simulink model "Modelo_Red_Mitigación_final"  (R2019b)
settings: Solver=VariableStepAuto  StartTime=0.0  StopTime=2.5  RelTol=1e-3
InitFcn:
  | Ts=20e-6;
undefined symbols (not defined in the file): D1, Delta, Ion, Lithium
libraries: powerlib x371, powerlib_meascontrol x286, simulink x50, simulink_extras x20, electricdrivelib x16
(part 7 of 11)

== system Modelo_Red_Mitigación_final/Modelo bateria pasiva/Subsystem3/Subsystem2 ==
  AC_CONTROL ALGORITHM : Subsystem
  Battery : electricdrivelib/Extra Sources/Battery  Commented=on  BatType=Lithium-Ion  ShowTempParam=off  ThermalPreset=no  ShowAgeParam=off  NomV=2000  NomQ=2  SOC=100  Batt_Tr=2  PresetModel=on  MaxQ=2  MinV=1500  FullV=2327.9743  Dis_rate=0.86957  R=10  Normal_OP=1.8087  expZone="[2160.7717     0.09826087]"  current=[0.2 0.4 1]  Units=Time  Tci=20  NomT=20  T2=-30  MaxQ2=4.8  FullV2=7.1  Normal_OP2=5.655  expZone2="[6.58           1]"  Rca=0.6  ti=2000  Dp=0  Neq0=0  Tsim=1e6  Ta1=25  Qeol=5.4*0.9  Reol=0.013333*1.2  Char_age=[2000, 3000]  Dis_age=[2000, 3000]  N1=1500  N2=10500  N3=1000  N4=1400  Ta2=45  N5=950
      settings: SourceProductName=Simscape Electrical
  Battery1 : electricdrivelib/Extra Sources/Battery  BatType=Lithium-Ion  ShowTempParam=off  ThermalPreset=no  ShowAgeParam=off  NomV=1800  NomQ=200  SOC=100  Batt_Tr=20  PresetModel=off  MaxQ=1  MinV=1500  FullV=2000  Dis_rate=5  R=0.1  Normal_OP=1  expZone="[1960.7717       0.9826087]"  current=[6.5 13 200]  Units=Time  Tci=20  NomT=20  T2=25  MaxQ2=200  FullV2=2000  Normal_OP2=1500  expZone2="[2160.7717       9.826087]"  Rca=0.6411  ti=4880  Dp=0  Neq0=0  Tsim=1e6  Ta1=25  Qeol=5.4*0.9  Reol=0.013333*1.2  Char_age=[2.3478, 3]  Dis_age=[2.3478, 10]  N1=1500  N2=10500  N3=1000  N4=1400  Ta2=45  N5=950
      settings: SourceProductName=Simscape Electrical
  Bus Selector : BusSelector  OutputSignals=SOC (%),Current (A),Voltage (V)
  Control1 : Subsystem
  "Control1 " : Subsystem  Commented=on
  Control2 : Subsystem  Commented=on
  Current Measurement1 : powerlib/Measurements/Current Measurement  PhasorSimulation=off  OutputType=Complex  PSBequivalent=0
      settings: SourceProductName=Simscape Electrical
  Current Measurement3 : powerlib/Measurements/Current Measurement  PhasorSimulation=off  OutputType=Complex  PSBequivalent=0
      settings: SourceProductName=Simscape Electrical
  Currents : Scope  NumInputPorts=2
  First-Order Filter3 : powerlib_meascontrol/Filters/First-Order Filter  FilterType=Lowpass  Tc=10e-3  Ts=0  Initialize=on  Vac_Init=[0, 0, 60]  Vdc_Init=0  PlotResponse=off  FreqRange="[0,  200,  1]"
      settings: SourceProductName=Simscape Electrical
  First-Order Filter4 : powerlib_meascontrol/Filters/First-Order Filter  FilterType=Lowpass  Tc=10e-3  Ts=0  Initialize=on  Vac_Init=[0, 0, 60]  Vdc_Init=0  PlotResponse=off  FreqRange="[0,  200,  1]"
      settings: SourceProductName=Simscape Electrical
  Half-Bridge Converter : powerlib/Power Electronics/Half-Bridge Converter  Commented=on  ModelType=Switching devices  Ron=1e-3  Rs=1e6  Cs=inf  Vforward=[0,0]  Ron_Diode=1e-3  Rs_Diode=1e6  Cs_Diode=inf  Vf_Diode=1e-3  Rs_CurrentSource=inf
      settings: SourceProductName=Simscape Electrical  SourceProductBaseCode=PS
  P SC in 1 : Scope
  "Power (3ph, Instantaneous)2" : powerlib_meascontrol/Measurements/Power (3ph, Instantaneous)
      settings: SourceProductName=Simscape Electrical
  Q Sc in 1 : Scope
  Series RLC Branch1 : powerlib/Elements/Series RLC Branch  LConnTagsString=__new0  RConnTagsString=__new0  BranchType=R  Resistance=0.1  Inductance=1e-3  SetiL0=off  InitialCurrent=0  Capacitance=220e-6  Setx0=off  InitialVoltage=0  Measurements=None
      settings: SourceProductName=Simscape Electrical
  Series RLC Branch2 : powerlib/Elements/Series RLC Branch  LConnTagsString=__new0  RConnTagsString=__new0  BranchType=C  Resistance=10e6  Inductance=1e-3  SetiL0=off  InitialCurrent=0  Capacitance=220e-6  Setx0=off  InitialVoltage=0  Measurements=None
      settings: SourceProductName=Simscape Electrical
  Series RLC Branch3 : powerlib/Elements/Series RLC Branch  LConnTagsString=__new0  RConnTagsString=__new0  BranchType=R  Resistance=0.5  Inductance=1e-3  SetiL0=off  InitialCurrent=0  Capacitance=220e-6  Setx0=off  InitialVoltage=0  Measurements=None
      settings: SourceProductName=Simscape Electrical
  Three-Phase V-I Measurement1 : powerlib/Measurements/Three-Phase V-I Measurement  VoltageMeasurement=phase-to-phase  SetLabelV=on  LabelV=Vabc_SC2  Vpu=off  VpuLL=off  CurrentMeasurement=yes  SetLabelI=on  LabelI=Iabc_SC2  Ipu=off  Pbase=100e6  Vbase=500e3  OutputType=Complex  PhasorSimulation=off  PSBequivalent=0
      settings: SourceProductName=Simscape Electrical
  To Workspace : ToWorkspace  VariableName=datosbatpasiva  SaveFormat=Timeseries  SampleTime=1E-5
  Two-Level Converter1 : powerlib/Power Electronics/Two-Level Converter  ModelType=Average model (Uref-controlled)  Ron=1e-3  Rs=1e6  Cs=inf  Vforward=[0,0]  Ron_Diode=1e-3  Rs_Diode=1e6  Cs_Diode=inf  Vf_Diode=1e-3  Rs_CurrentSource=inf
      settings: SourceProductName=Simscape Electrical  SourceProductBaseCode=PS
  V DC : Scope  NumInputPorts=2
  Variables SC1 : Scope  NumInputPorts=3
  VinvSC : Scope  NumInputPorts=2
  Voltage Measurement : powerlib/Measurements/Voltage Measurement  PhasorSimulation=off  OutputType=Complex  PSBequivalent=0
      settings: SourceProductName=Simscape Electrical
  A : PMIOPort  Side=Left
  B : PMIOPort  Port=2  Side=Left
  C : PMIOPort  Port=3  Side=Left
  tag scope: Iload=global, Vdc=global
  wires:
  [Iobat] -> Currents/2
  [Ibat] -> Currents/1  "Ibatout"
  Voltage Measurement/1 -> [Vdc]
  Current Measurement1/1 -> [Iload]
  Current Measurement3/1 -> [Iobat]
  [IoutConv] -> V DC/2
  [Vdc] -> V DC/1
  [Uref] -> Two-Level Converter1/1
  [Vabc_SC2] -> VinvSC/1
  "Power (3ph, Instantaneous)2"/1 -> First-Order Filter3/1
  First-Order Filter4/1 -> Q Sc in 1/1
  [Vabc_SC2] -> "Power (3ph, Instantaneous)2"/1
  First-Order Filter3/1 -> P SC in 1/1
  [Iabc_SC2] -> "Power (3ph, Instantaneous)2"/2
  "Power (3ph, Instantaneous)2"/2 -> First-Order Filter4/1
  Battery1/1 -> Bus Selector/1, To Workspace/1
  Bus Selector/1 -> Variables SC1/1  "<SOC (%)>"
  Bus Selector/3 -> Variables SC1/3  "<Voltage (V)>"
  Bus Selector/2 -> Variables SC1/2  "<Current (A)>"
  connections:
  Voltage Measurement/LConn1 -- Current Measurement3/RConn1 -- Series RLC Branch2/LConn1 -- Current Measurement1/LConn1
  Current Measurement1/RConn1 -- Two-Level Converter1/RConn1
  A/RConn1 -- Three-Phase V-I Measurement1/LConn1
  C/RConn1 -- Three-Phase V-I Measurement1/LConn3
  B/RConn1 -- Three-Phase V-I Measurement1/LConn2
  Three-Phase V-I Measurement1/RConn1 -- Two-Level Converter1/LConn1
  Three-Phase V-I Measurement1/RConn2 -- Two-Level Converter1/LConn2
  Three-Phase V-I Measurement1/RConn3 -- Two-Level Converter1/LConn3
  Voltage Measurement/LConn2 -- Battery1/LConn2 -- Series RLC Branch3/RConn1 -- Two-Level Converter1/RConn2 -- Series RLC Branch2/RConn1
  Series RLC Branch1/LConn1 -- Current Measurement3/LConn1
  Series RLC Branch1/RConn1 -- Battery1/LConn1 -- Series RLC Branch3/LConn1

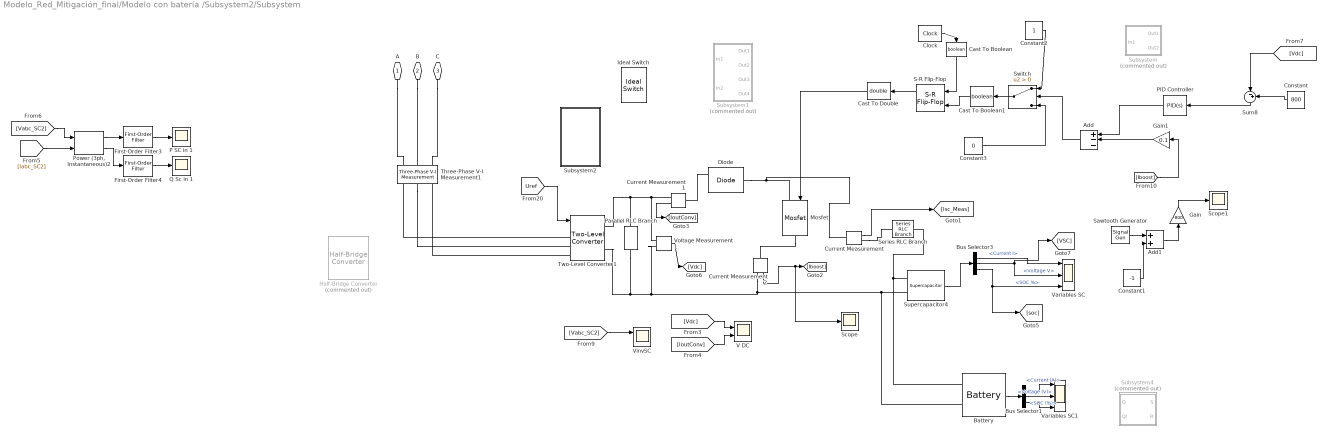
== system Modelo_Red_Mitigación_final/Modelo con batería /Subsystem2/Subsystem ==
  Add : Sum  Inputs=+--
  Add1 : Sum
  Battery : electricdrivelib/Extra Sources/Battery  BatType=Lithium-Ion  ShowTempParam=off  ThermalPreset=no  ShowAgeParam=off  NomV=500  NomQ=500  SOC=100  Batt_Tr=30  PresetModel=on  MaxQ=500  MinV=375  FullV=581.9936  Dis_rate=217.3913  R=0.01  Normal_OP=452.1739  expZone="[540.1929      24.56522]"  current=[6.5 13 32.5]  Units=Time  Tci=20  NomT=20  T2=-30  MaxQ2=4.8  FullV2=7.1  Normal_OP2=5.655  expZone2="[6.58           1]"  Rca=0.6  ti=2000  Dp=0  Neq0=0  Tsim=1e6  Ta1=25  Qeol=5.4*0.9  Reol=0.013333*1.2  Char_age=[2.3478, 3]  Dis_age=[2.3478, 10]  N1=1500  N2=10500  N3=1000  N4=1400  Ta2=45  N5=950
      settings: SourceProductName=Simscape Electrical
  Bus Selector1 : BusSelector  OutputSignals=Current (A),Voltage (V),SOC (%)
  Bus Selector3 : BusSelector  OutputSignals=Current I,Voltage V,SOC %
  Cast To Boolean : DataTypeConversion  OutDataTypeStr=boolean
  Cast To Boolean1 : DataTypeConversion  OutDataTypeStr=boolean
  Cast To Double : DataTypeConversion  OutDataTypeStr=double
  Clock : simulink_extras/Flip Flops/Clock  period=1/10e3
  Constant : Constant  Value=800
  Constant1 : Constant  Value=-1
  Constant2 : Constant
  Constant3 : Constant  Value=0
  Current Measurement : powerlib/Measurements/Current Measurement  PhasorSimulation=off  OutputType=Complex  PSBequivalent=0
      settings: SourceProductName=Simscape Electrical
  Current Measurement1 : powerlib/Measurements/Current Measurement  PhasorSimulation=off  OutputType=Complex  PSBequivalent=0
      settings: SourceProductName=Simscape Electrical
  Current Measurement2 : powerlib/Measurements/Current Measurement  PhasorSimulation=off  OutputType=Complex  PSBequivalent=0
      settings: SourceProductName=Simscape Electrical
  Diode : powerlib/Power Electronics/Diode  Ron=0.001  Lon=0  Vf=0.8  IC=0  UseSnubber=0  Rs=500  Cs=250e-9  Measurements=on
      settings: SourceProductName=Simscape Electrical
  First-Order Filter3 : powerlib_meascontrol/Filters/First-Order Filter  FilterType=Lowpass  Tc=10e-3  Ts=0  Initialize=on  Vac_Init=[0, 0, 60]  Vdc_Init=0  PlotResponse=off  FreqRange="[0,  200,  1]"
      settings: SourceProductName=Simscape Electrical
  First-Order Filter4 : powerlib_meascontrol/Filters/First-Order Filter  FilterType=Lowpass  Tc=10e-3  Ts=0  Initialize=on  Vac_Init=[0, 0, 60]  Vdc_Init=0  PlotResponse=off  FreqRange="[0,  200,  1]"
      settings: SourceProductName=Simscape Electrical
  Gain : Gain  Gain=-800
  Gain1 : Gain  Gain=0.1
  Half-Bridge Converter : powerlib/Power Electronics/Half-Bridge Converter  Commented=on  ModelType=Switching devices  Ron=1e-3  Rs=1e6  Cs=inf  Vforward=[0,0]  Ron_Diode=1e-3  Rs_Diode=1e6  Cs_Diode=inf  Vf_Diode=1e-3  Rs_CurrentSource=inf
      settings: SourceProductName=Simscape Electrical  SourceProductBaseCode=PS
  Ideal Switch : powerlib/Power Electronics/Ideal Switch  Ron=1e-3  Lon=0  IC=1  Rs=1e5  Cs=inf  Measurements=on
      settings: SourceProductName=Simscape Electrical
  Mosfet : powerlib/Power Electronics/Mosfet  Ron=0.1  Lon=0  Rd=0.01  Vfd=0  IC=0  Rs=1e5  Cs=inf  Measurements=off
      settings: SourceProductName=Simscape Electrical
  P SC in 1 : Scope
  PID Controller : simulink/Continuous/PID Controller  Controller=PID  Form=Parallel  TimeDomain=Continuous-time  SampleTime=-1  IntegratorMethod=Forward Euler  FilterMethod=Forward Euler  ControllerParametersSource=internal  P=40  I=10  D=0  UseFilter=on  N=100  TunerSelectOption=Transfer Function Based (PID Tuner App)  InitialConditionSource=internal  InitialConditionForIntegrator=0  InitialConditionForFilter=0  DifferentiatorICPrevScaledInput=0  ExternalReset=none  TrackingMode=off  Kt=1  LimitOutput=off  UpperSaturationLimit=inf  LowerSaturationLimit=-inf  LinearizeAsGain=on  AntiWindupMode=none  Kb=1  POutMin=[]  POutMax=[]  IOutMin=[]  IOutMax=[]  DOutMin=[]  DOutMax=[]  NOutMin=[]  NOutMax=[]  SumOutMin=[]  SumOutMax=[]  SaturationOutMin=[]  SaturationOutMax=[]  PParamMin=[]  PParamMax=[]  IParamMin=[]  IParamMax=[]  DParamMin=[]  DParamMax=[]  NParamMin=[]  NParamMax=[]  KbParamMin=[]  KbParamMax=[]  KtParamMin=[]  KtParamMax=[]  KbOutMin=[]  KbOutMax=[]  KtOutMin=[]  KtOutMax=[]  IntegratorOutMin=[]  IntegratorOutMax=[]  FilterOutMin=[]  FilterOutMax=[]  SumI1OutMin=[]  SumI1OutMax=[]  SumI2OutMin=[]  SumI2OutMax=[]  SumI3OutMin=[]  SumI3OutMax=[]  SumI4OutMin=[]  SumI4OutMax=[]  SumDOutMin=[]  SumDOutMax=[]  DifferentiatorOutMin=[]  DifferentiatorOutMax=[]  FilterDiffOutCoefMin=[]  FilterDiffOutCoefMax=[]  ReciprocalOutMin=[]  ReciprocalOutMax=[]  SumDenOutMin=[]  SumDenOutMax=[]  SumNumOutMin=[]  SumNumOutMax=[]  DivideOutMin=[]  DivideOutMax=[]  IntegratorContinuousStateAttributes=''  IntegratorStateMustResolveToSignalObject=off  IntegratorRTWStateStorageClass=Auto  FilterContinuousStateAttributes=''  FilterStateMustResolveToSignalObject=off  FilterRTWStateStorageClass=Auto  ParallelPVariant=InternalParameters  IdealPVariant=Disabled  IVariant=InternalParameters  DVariant=InternalParameters  IntegratorVariant=Continuous  SatVariant=Disabled  AWVariant=Passthrough  PCopyVariant=Disabled  TRVariant=Disabled  FdbkBlocksVariant=Forward  IdealPFdbkVariant=Disabled  SatFdbkVariant=Disabled  DerivativeFilterVariant=ContFilter  NVariant=InternalParameters  NCopyVariant=Disabled  FilterICVariant=InternalICsFilter  IntegratorICVariant=InternalICs  ExternalResetVariant=Disabled  TRSumVariant=Passthrough  SumFdbkVariant=Disabled  SumVariant=Sum_PID
  Parallel RLC Branch : powerlib/Elements/Parallel RLC Branch  LConnTagsString=a  RConnTagsString=__new0  BranchType=C  Resistance=0.01  Inductance=1e-3  SetiL0=off  InitialCurrent=0  Capacitance=6600e-6  Setx0=off  InitialVoltage=800  Measurements=None
      settings: SourceProductName=Simscape Electrical
  "Power (3ph, Instantaneous)2" : powerlib_meascontrol/Measurements/Power (3ph, Instantaneous)
      settings: SourceProductName=Simscape Electrical
  Q Sc in 1 : Scope
  S-R Flip-Flop : simulink_extras/Flip Flops/S-R Flip-Flop  initial_condition=1
  Sawtooth Generator : SignalGenerator  WaveForm=sawtooth  Frequency=10e3
  Scope : Scope
  Scope1 : Scope
  Series RLC Branch : powerlib/Elements/Series RLC Branch  LConnTagsString=__new0  RConnTagsString=__new0  BranchType=L  Resistance=65e-3  Inductance=1e-3  SetiL0=off  InitialCurrent=0  Capacitance=1e-6  Setx0=off  InitialVoltage=0  Measurements=None
      settings: SourceProductName=Simscape Electrical
  Subsystem : Subsystem  Commented=on
  Subsystem1 : Subsystem  Commented=on
  Subsystem2 : Subsystem
  Subsystem4 : Subsystem  Commented=on
  Sum8 : Sum  Inputs=|-+
  Supercapacitor4 : electricdrivelib/Extra Sources/Supercapacitor  C=18  Rdc=7e-3  Voltage=500  Ns=1  Np=1  Vinit=500  Temp=25  PresetModel=on  EstParam=off  Nc=1  r=1e-9  epsilon=6.0208e-10  Ich=10  Vstern="[0.161  2.7  7.8]"  Self_dis=off  Ioc=10  Vself="[48  47.8  47.06  44.65]"  demandeplot=off  I="[10  20 100  500]"  Units=sec  Vmax=0  If=0  deltaV=0  alpha=0  sec=0
      settings: SourceProductName=Simscape Electrical  SourceProductBaseCode=PS
  Switch : Switch  Criteria=u2 > Threshold
  Three-Phase V-I Measurement1 : powerlib/Measurements/Three-Phase V-I Measurement  VoltageMeasurement=phase-to-phase  SetLabelV=on  LabelV=Vabc_SC2  Vpu=off  VpuLL=off  CurrentMeasurement=yes  SetLabelI=on  LabelI=Iabc_SC2  Ipu=off  Pbase=100e6  Vbase=500e3  OutputType=Complex  PhasorSimulation=off  PSBequivalent=0
      settings: SourceProductName=Simscape Electrical
  Two-Level Converter1 : powerlib/Power Electronics/Two-Level Converter  ModelType=Average model (Uref-controlled)  Ron=1e-3  Rs=1e6  Cs=inf  Vforward=[0,0]  Ron_Diode=1e-3  Rs_Diode=1e6  Cs_Diode=inf  Vf_Diode=1e-3  Rs_CurrentSource=inf
      settings: SourceProductName=Simscape Electrical  SourceProductBaseCode=PS
  V DC : Scope  NumInputPorts=2
  Variables SC : Scope  NumInputPorts=3
  Variables SC1 : Scope  NumInputPorts=3
  VinvSC : Scope  NumInputPorts=2
  Voltage Measurement1 : powerlib/Measurements/Voltage Measurement  PhasorSimulation=off  OutputType=Complex  PSBequivalent=0
      settings: SourceProductName=Simscape Electrical
  A : PMIOPort  Side=Left
  B : PMIOPort  Port=2  Side=Left
  C : PMIOPort  Port=3  Side=Left
  wires:
  Current Measurement/1 -> [Isc_Meas]
  Bus Selector3/2 -> Variables SC/2, [VSC]  "<Voltage V>"
  Bus Selector3/3 -> [soc], Variables SC/3  "<SOC %>"
  Bus Selector3/1 -> Variables SC/1  "<Current I>"
  "Power (3ph, Instantaneous)2"/2 -> First-Order Filter4/1
  [Iabc_SC2] -> "Power (3ph, Instantaneous)2"/2
  First-Order Filter3/1 -> P SC in 1/1
  [Vabc_SC2] -> "Power (3ph, Instantaneous)2"/1
  First-Order Filter4/1 -> Q Sc in 1/1
  "Power (3ph, Instantaneous)2"/1 -> First-Order Filter3/1
  [Vabc_SC2] -> VinvSC/1
  Voltage Measurement1/1 -> [Vdc]
  [Uref] -> Two-Level Converter1/1
  Current Measurement1/1 -> [IoutConv]
  [Vdc] -> V DC/1
  [IoutConv] -> V DC/2
  Supercapacitor4/1 -> Bus Selector3/1
  Current Measurement2/1 -> Scope/1, [Iboost]
  [Iboost] -> Gain1/1
  Constant/1 -> Sum8/2
  [Vdc] -> Sum8/1
  Cast To Boolean1/1 -> S-R Flip-Flop/2
  Cast To Double/1 -> Mosfet/1
  Clock/1 -> Cast To Boolean/1
  Add/1 -> Switch/2
  Cast To Boolean/1 -> S-R Flip-Flop/1
  S-R Flip-Flop/1 -> Cast To Double/1
  Constant3/1 -> Switch/3
  Switch/1 -> Cast To Boolean1/1
  Constant2/1 -> Switch/1
  Sum8/1 -> PID Controller/1
  Bus Selector1/2 -> Variables SC1/2  "<Voltage (V)>"
  Battery/1 -> Bus Selector1/1
  Bus Selector1/3 -> Variables SC1/3  "<SOC (%)>"
  Bus Selector1/1 -> Variables SC1/1  "<Current (A)>"
  Gain1/1 -> Add/2
  PID Controller/1 -> Add/1
  Sawtooth Generator/1 -> Add1/1
  Add1/1 -> Gain/1
  Constant1/1 -> Add1/2
  Gain/1 -> Scope1/1
  connections:
  Current Measurement/RConn1 -- Series RLC Branch/LConn1
  Voltage Measurement1/LConn2 -- Battery/LConn2 -- Supercapacitor4/LConn2 -- Current Measurement2/RConn1 -- Two-Level Converter1/RConn2 -- Parallel RLC Branch/RConn1
  B/RConn1 -- Three-Phase V-I Measurement1/LConn2
  C/RConn1 -- Three-Phase V-I Measurement1/LConn3
  A/RConn1 -- Three-Phase V-I Measurement1/LConn1
  Parallel RLC Branch/LConn1 -- Two-Level Converter1/RConn1 -- Current Measurement1/RConn1 -- Voltage Measurement1/LConn1
  Diode/LConn1 -- Mosfet/LConn1 -- Current Measurement/LConn1
  Two-Level Converter1/LConn1 -- Three-Phase V-I Measurement1/RConn1
  Three-Phase V-I Measurement1/RConn2 -- Two-Level Converter1/LConn2
  Two-Level Converter1/LConn3 -- Three-Phase V-I Measurement1/RConn3
  Mosfet/RConn1 -- Current Measurement2/LConn1
  Diode/RConn1 -- Current Measurement1/LConn1
  Supercapacitor4/LConn1 -- Battery/LConn1 -- Series RLC Branch/RConn1

== system Modelo_Red_Mitigación_final/Modelo con batería /Subsystem3/Subsystem2 ==
  AC_CONTROL ALGORITHM : Subsystem
  Battery : electricdrivelib/Extra Sources/Battery  BatType=Lithium-Ion  ShowTempParam=off  ThermalPreset=no  ShowAgeParam=off  NomV=1000  NomQ=10  SOC=80  Batt_Tr=2  PresetModel=on  MaxQ=10  MinV=750  FullV=1163.9871  Dis_rate=4.3478  R=1  Normal_OP=9.0435  expZone="[1080.3859     0.49130435]"  current=[0.2 0.4 1]  Units=Time  Tci=20  NomT=20  T2=-30  MaxQ2=4.8  FullV2=7.1  Normal_OP2=5.655  expZone2="[6.58           1]"  Rca=0.6  ti=2000  Dp=0  Neq0=0  Tsim=1e6  Ta1=25  Qeol=5.4*0.9  Reol=0.013333*1.2  Char_age=[2000, 3000]  Dis_age=[2000, 3000]  N1=1500  N2=10500  N3=1000  N4=1400  Ta2=45  N5=950
      settings: SourceProductName=Simscape Electrical
  Bus Selector1 : BusSelector  OutputSignals=Current (A),Voltage (V),SOC (%)
  Control1 : Subsystem
  "Control1 " : Subsystem  Commented=on
  Control2 : Subsystem  Commented=on
  Current Measurement1 : powerlib/Measurements/Current Measurement  PhasorSimulation=off  OutputType=Complex  PSBequivalent=0
      settings: SourceProductName=Simscape Electrical
  Current Measurement2 : powerlib/Measurements/Current Measurement  PhasorSimulation=off  OutputType=Complex  PSBequivalent=0
      settings: SourceProductName=Simscape Electrical
  Current Measurement3 : powerlib/Measurements/Current Measurement  PhasorSimulation=off  OutputType=Complex  PSBequivalent=0
      settings: SourceProductName=Simscape Electrical
  Currents : Scope  NumInputPorts=2
  First-Order Filter3 : powerlib_meascontrol/Filters/First-Order Filter  FilterType=Lowpass  Tc=10e-3  Ts=0  Initialize=on  Vac_Init=[0, 0, 60]  Vdc_Init=0  PlotResponse=off  FreqRange="[0,  200,  1]"
      settings: SourceProductName=Simscape Electrical
  First-Order Filter4 : powerlib_meascontrol/Filters/First-Order Filter  FilterType=Lowpass  Tc=10e-3  Ts=0  Initialize=on  Vac_Init=[0, 0, 60]  Vdc_Init=0  PlotResponse=off  FreqRange="[0,  200,  1]"
      settings: SourceProductName=Simscape Electrical
  Ground : powerlib/Elements/Ground  LConnTagsString=a
      settings: SourceProductName=Simscape Electrical
  Half-Bridge Converter : powerlib/Power Electronics/Half-Bridge Converter  Commented=on  ModelType=Switching devices  Ron=1e-3  Rs=1e6  Cs=inf  Vforward=[0,0]  Ron_Diode=1e-3  Rs_Diode=1e6  Cs_Diode=inf  Vf_Diode=1e-3  Rs_CurrentSource=inf
      settings: SourceProductName=Simscape Electrical  SourceProductBaseCode=PS
  Half-Bridge Converter2 : powerlib/Power Electronics/Half-Bridge Converter  ModelType=Switching devices  Ron=1e-3  Rs=1e6  Cs=inf  Vforward=[0,0]  Ron_Diode=1e-3  Rs_Diode=1e6  Cs_Diode=inf  Vf_Diode=1e-3  Rs_CurrentSource=inf
      settings: SourceProductName=Simscape Electrical  SourceProductBaseCode=PS
  P SC in 1 : Scope
  Parallel RLC Branch : powerlib/Elements/Parallel RLC Branch  LConnTagsString=a  RConnTagsString=__new0  BranchType=C  Resistance=0.01  Inductance=1e-3  SetiL0=off  InitialCurrent=0  Capacitance=220e-6  Setx0=on  InitialVoltage=1500  Measurements=None
      settings: SourceProductName=Simscape Electrical
  "Power (3ph, Instantaneous)2" : powerlib_meascontrol/Measurements/Power (3ph, Instantaneous)
      settings: SourceProductName=Simscape Electrical
  Q Sc in 1 : Scope
  Series RLC Branch1 : powerlib/Elements/Series RLC Branch  LConnTagsString=__new0  RConnTagsString=__new0  BranchType=L  Resistance=65e-3  Inductance=1.67e-3  SetiL0=off  InitialCurrent=0  Capacitance=1e-6  Setx0=off  InitialVoltage=0  Measurements=None
      settings: SourceProductName=Simscape Electrical
  Three-Phase V-I Measurement1 : powerlib/Measurements/Three-Phase V-I Measurement  VoltageMeasurement=phase-to-phase  SetLabelV=on  LabelV=Vabc_SC2  Vpu=off  VpuLL=off  CurrentMeasurement=yes  SetLabelI=on  LabelI=Iabc_SC2  Ipu=off  Pbase=100e6  Vbase=500e3  OutputType=Complex  PhasorSimulation=off  PSBequivalent=0
      settings: SourceProductName=Simscape Electrical
  Two-Level Converter1 : powerlib/Power Electronics/Two-Level Converter  ModelType=Average model (Uref-controlled)  Ron=1e-3  Rs=1e6  Cs=inf  Vforward=[0,0]  Ron_Diode=1e-3  Rs_Diode=1e6  Cs_Diode=inf  Vf_Diode=1e-3  Rs_CurrentSource=inf
      settings: SourceProductName=Simscape Electrical  SourceProductBaseCode=PS
  V DC : Scope  NumInputPorts=2
  Variables SC1 : Scope  NumInputPorts=3
  VinvSC : Scope  NumInputPorts=2
  Voltage Measurement : powerlib/Measurements/Voltage Measurement  PhasorSimulation=off  OutputType=Complex  PSBequivalent=0
      settings: SourceProductName=Simscape Electrical
  A : PMIOPort  Side=Left
  B : PMIOPort  Port=2  Side=Left
  C : PMIOPort  Port=3  Side=Left
  tag scope: Ibat=global, Iload=global, Iobat=global, Vdc=global
  wires:
  "Power (3ph, Instantaneous)2"/2 -> First-Order Filter4/1
  [Iabc_SC2] -> "Power (3ph, Instantaneous)2"/2
  First-Order Filter3/1 -> P SC in 1/1
  [Vabc_SC2] -> "Power (3ph, Instantaneous)2"/1
  First-Order Filter4/1 -> Q Sc in 1/1
  "Power (3ph, Instantaneous)2"/1 -> First-Order Filter3/1
  [Vabc_SC2] -> VinvSC/1
  [Uref] -> Two-Level Converter1/1
  [Vdc] -> V DC/1
  [IoutConv] -> V DC/2
  Bus Selector1/2 -> Variables SC1/2  "<Voltage (V)>"
  Battery/1 -> Bus Selector1/1
  Bus Selector1/3 -> Variables SC1/3  "<SOC (%)>"
  Bus Selector1/1 -> Variables SC1/1  "<Current (A)>"
  Current Measurement1/1 -> [Iload]
  Voltage Measurement/1 -> [Vdc]
  [G_BAT] -> Half-Bridge Converter2/1
  Current Measurement3/1 -> [Iobat]
  [Ibat] -> Currents/1  "Ibatout"
  Current Measurement2/1 -> [Ibat]
  [Iobat] -> Currents/2
  connections:
  B/RConn1 -- Three-Phase V-I Measurement1/LConn2
  C/RConn1 -- Three-Phase V-I Measurement1/LConn3
  A/RConn1 -- Three-Phase V-I Measurement1/LConn1
  Two-Level Converter1/LConn1 -- Three-Phase V-I Measurement1/RConn1
  Three-Phase V-I Measurement1/RConn2 -- Two-Level Converter1/LConn2
  Two-Level Converter1/LConn3 -- Three-Phase V-I Measurement1/RConn3
  Half-Bridge Converter2/RConn2 -- Battery/LConn2 -- Ground/LConn1 -- Two-Level Converter1/RConn2 -- Parallel RLC Branch/RConn1 -- Voltage Measurement/LConn2
  Battery/LConn1 -- Series RLC Branch1/RConn1
  Current Measurement1/RConn1 -- Two-Level Converter1/RConn1
  Current Measurement3/LConn1 -- Half-Bridge Converter2/RConn1
  Current Measurement2/LConn1 -- Series RLC Branch1/LConn1
  Current Measurement2/RConn1 -- Half-Bridge Converter2/LConn1
  Parallel RLC Branch/LConn1 -- Current Measurement3/RConn1 -- Voltage Measurement/LConn1 -- Current Measurement1/LConn1

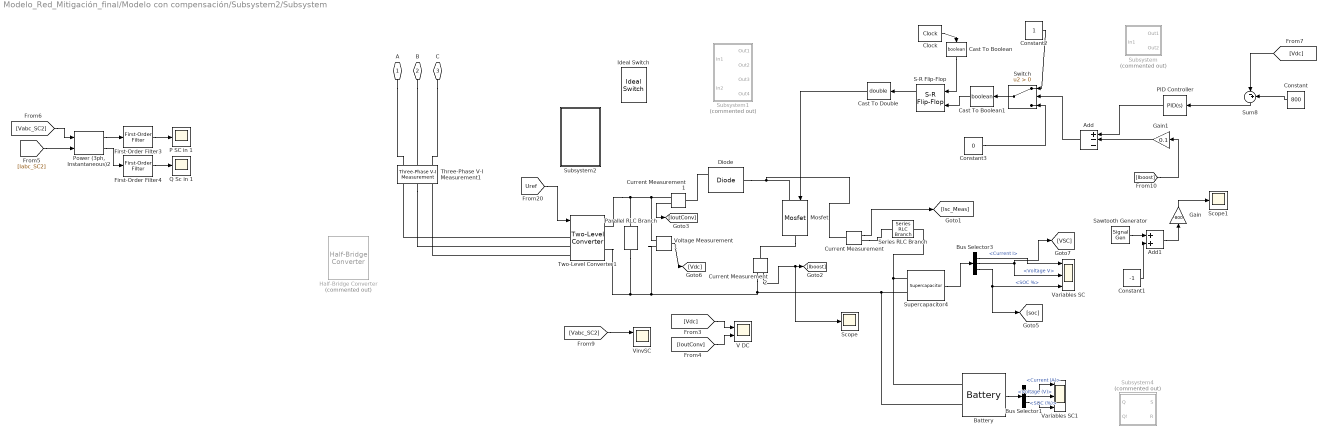
== system Modelo_Red_Mitigación_final/Modelo con compensación/Subsystem2/Subsystem ==
  Add : Sum  Inputs=+--
  Add1 : Sum
  Battery : electricdrivelib/Extra Sources/Battery  BatType=Lithium-Ion  ShowTempParam=off  ThermalPreset=no  ShowAgeParam=off  NomV=500  NomQ=500  SOC=100  Batt_Tr=30  PresetModel=on  MaxQ=500  MinV=375  FullV=581.9936  Dis_rate=217.3913  R=0.01  Normal_OP=452.1739  expZone="[540.1929      24.56522]"  current=[6.5 13 32.5]  Units=Time  Tci=20  NomT=20  T2=-30  MaxQ2=4.8  FullV2=7.1  Normal_OP2=5.655  expZone2="[6.58           1]"  Rca=0.6  ti=2000  Dp=0  Neq0=0  Tsim=1e6  Ta1=25  Qeol=5.4*0.9  Reol=0.013333*1.2  Char_age=[2.3478, 3]  Dis_age=[2.3478, 10]  N1=1500  N2=10500  N3=1000  N4=1400  Ta2=45  N5=950
      settings: SourceProductName=Simscape Electrical
  Bus Selector1 : BusSelector  OutputSignals=Current (A),Voltage (V),SOC (%)
  Bus Selector3 : BusSelector  OutputSignals=Current I,Voltage V,SOC %
  Cast To Boolean : DataTypeConversion  OutDataTypeStr=boolean
  Cast To Boolean1 : DataTypeConversion  OutDataTypeStr=boolean
  Cast To Double : DataTypeConversion  OutDataTypeStr=double
  Clock : simulink_extras/Flip Flops/Clock  period=1/10e3
  Constant : Constant  Value=800
  Constant1 : Constant  Value=-1
  Constant2 : Constant
  Constant3 : Constant  Value=0
  Current Measurement : powerlib/Measurements/Current Measurement  PhasorSimulation=off  OutputType=Complex  PSBequivalent=0
      settings: SourceProductName=Simscape Electrical
  Current Measurement1 : powerlib/Measurements/Current Measurement  PhasorSimulation=off  OutputType=Complex  PSBequivalent=0
      settings: SourceProductName=Simscape Electrical
  Current Measurement2 : powerlib/Measurements/Current Measurement  PhasorSimulation=off  OutputType=Complex  PSBequivalent=0
      settings: SourceProductName=Simscape Electrical
  Diode : powerlib/Power Electronics/Diode  Ron=0.001  Lon=0  Vf=0.8  IC=0  UseSnubber=0  Rs=500  Cs=250e-9  Measurements=on
      settings: SourceProductName=Simscape Electrical
  First-Order Filter3 : powerlib_meascontrol/Filters/First-Order Filter  FilterType=Lowpass  Tc=10e-3  Ts=0  Initialize=on  Vac_Init=[0, 0, 60]  Vdc_Init=0  PlotResponse=off  FreqRange="[0,  200,  1]"
      settings: SourceProductName=Simscape Electrical
  First-Order Filter4 : powerlib_meascontrol/Filters/First-Order Filter  FilterType=Lowpass  Tc=10e-3  Ts=0  Initialize=on  Vac_Init=[0, 0, 60]  Vdc_Init=0  PlotResponse=off  FreqRange="[0,  200,  1]"
      settings: SourceProductName=Simscape Electrical
  Gain : Gain  Gain=-800
  Gain1 : Gain  Gain=0.1
  Half-Bridge Converter : powerlib/Power Electronics/Half-Bridge Converter  Commented=on  ModelType=Switching devices  Ron=1e-3  Rs=1e6  Cs=inf  Vforward=[0,0]  Ron_Diode=1e-3  Rs_Diode=1e6  Cs_Diode=inf  Vf_Diode=1e-3  Rs_CurrentSource=inf
      settings: SourceProductName=Simscape Electrical  SourceProductBaseCode=PS
  Ideal Switch : powerlib/Power Electronics/Ideal Switch  Ron=1e-3  Lon=0  IC=1  Rs=1e5  Cs=inf  Measurements=on
      settings: SourceProductName=Simscape Electrical
  Mosfet : powerlib/Power Electronics/Mosfet  Ron=0.1  Lon=0  Rd=0.01  Vfd=0  IC=0  Rs=1e5  Cs=inf  Measurements=off
      settings: SourceProductName=Simscape Electrical
  P SC in 1 : Scope
  PID Controller : simulink/Continuous/PID Controller  Controller=PID  Form=Parallel  TimeDomain=Continuous-time  SampleTime=-1  IntegratorMethod=Forward Euler  FilterMethod=Forward Euler  ControllerParametersSource=internal  P=40  I=10  D=0  UseFilter=on  N=100  TunerSelectOption=Transfer Function Based (PID Tuner App)  InitialConditionSource=internal  InitialConditionForIntegrator=0  InitialConditionForFilter=0  DifferentiatorICPrevScaledInput=0  ExternalReset=none  TrackingMode=off  Kt=1  LimitOutput=off  UpperSaturationLimit=inf  LowerSaturationLimit=-inf  LinearizeAsGain=on  AntiWindupMode=none  Kb=1  POutMin=[]  POutMax=[]  IOutMin=[]  IOutMax=[]  DOutMin=[]  DOutMax=[]  NOutMin=[]  NOutMax=[]  SumOutMin=[]  SumOutMax=[]  SaturationOutMin=[]  SaturationOutMax=[]  PParamMin=[]  PParamMax=[]  IParamMin=[]  IParamMax=[]  DParamMin=[]  DParamMax=[]  NParamMin=[]  NParamMax=[]  KbParamMin=[]  KbParamMax=[]  KtParamMin=[]  KtParamMax=[]  KbOutMin=[]  KbOutMax=[]  KtOutMin=[]  KtOutMax=[]  IntegratorOutMin=[]  IntegratorOutMax=[]  FilterOutMin=[]  FilterOutMax=[]  SumI1OutMin=[]  SumI1OutMax=[]  SumI2OutMin=[]  SumI2OutMax=[]  SumI3OutMin=[]  SumI3OutMax=[]  SumI4OutMin=[]  SumI4OutMax=[]  SumDOutMin=[]  SumDOutMax=[]  DifferentiatorOutMin=[]  DifferentiatorOutMax=[]  FilterDiffOutCoefMin=[]  FilterDiffOutCoefMax=[]  ReciprocalOutMin=[]  ReciprocalOutMax=[]  SumDenOutMin=[]  SumDenOutMax=[]  SumNumOutMin=[]  SumNumOutMax=[]  DivideOutMin=[]  DivideOutMax=[]  IntegratorContinuousStateAttributes=''  IntegratorStateMustResolveToSignalObject=off  IntegratorRTWStateStorageClass=Auto  FilterContinuousStateAttributes=''  FilterStateMustResolveToSignalObject=off  FilterRTWStateStorageClass=Auto  ParallelPVariant=InternalParameters  IdealPVariant=Disabled  IVariant=InternalParameters  DVariant=InternalParameters  IntegratorVariant=Continuous  SatVariant=Disabled  AWVariant=Passthrough  PCopyVariant=Disabled  TRVariant=Disabled  FdbkBlocksVariant=Forward  IdealPFdbkVariant=Disabled  SatFdbkVariant=Disabled  DerivativeFilterVariant=ContFilter  NVariant=InternalParameters  NCopyVariant=Disabled  FilterICVariant=InternalICsFilter  IntegratorICVariant=InternalICs  ExternalResetVariant=Disabled  TRSumVariant=Passthrough  SumFdbkVariant=Disabled  SumVariant=Sum_PID
  Parallel RLC Branch : powerlib/Elements/Parallel RLC Branch  LConnTagsString=a  RConnTagsString=__new0  BranchType=C  Resistance=0.01  Inductance=1e-3  SetiL0=off  InitialCurrent=0  Capacitance=6600e-6  Setx0=off  InitialVoltage=800  Measurements=None
      settings: SourceProductName=Simscape Electrical
  "Power (3ph, Instantaneous)2" : powerlib_meascontrol/Measurements/Power (3ph, Instantaneous)
      settings: SourceProductName=Simscape Electrical
  Q Sc in 1 : Scope
  S-R Flip-Flop : simulink_extras/Flip Flops/S-R Flip-Flop  initial_condition=1
  Sawtooth Generator : SignalGenerator  WaveForm=sawtooth  Frequency=10e3
  Scope : Scope
  Scope1 : Scope
  Series RLC Branch : powerlib/Elements/Series RLC Branch  LConnTagsString=__new0  RConnTagsString=__new0  BranchType=L  Resistance=65e-3  Inductance=1e-3  SetiL0=off  InitialCurrent=0  Capacitance=1e-6  Setx0=off  InitialVoltage=0  Measurements=None
      settings: SourceProductName=Simscape Electrical
  Subsystem : Subsystem  Commented=on
  Subsystem1 : Subsystem  Commented=on
  Subsystem2 : Subsystem
  Subsystem4 : Subsystem  Commented=on
  Sum8 : Sum  Inputs=|-+
  Supercapacitor4 : electricdrivelib/Extra Sources/Supercapacitor  C=18  Rdc=7e-3  Voltage=500  Ns=1  Np=1  Vinit=500  Temp=25  PresetModel=on  EstParam=off  Nc=1  r=1e-9  epsilon=6.0208e-10  Ich=10  Vstern="[0.161  2.7  7.8]"  Self_dis=off  Ioc=10  Vself="[48  47.8  47.06  44.65]"  demandeplot=off  I="[10  20 100  500]"  Units=sec  Vmax=0  If=0  deltaV=0  alpha=0  sec=0
      settings: SourceProductName=Simscape Electrical  SourceProductBaseCode=PS
  Switch : Switch  Criteria=u2 > Threshold
  Three-Phase V-I Measurement1 : powerlib/Measurements/Three-Phase V-I Measurement  VoltageMeasurement=phase-to-phase  SetLabelV=on  LabelV=Vabc_SC2  Vpu=off  VpuLL=off  CurrentMeasurement=yes  SetLabelI=on  LabelI=Iabc_SC2  Ipu=off  Pbase=100e6  Vbase=500e3  OutputType=Complex  PhasorSimulation=off  PSBequivalent=0
      settings: SourceProductName=Simscape Electrical
  Two-Level Converter1 : powerlib/Power Electronics/Two-Level Converter  ModelType=Average model (Uref-controlled)  Ron=1e-3  Rs=1e6  Cs=inf  Vforward=[0,0]  Ron_Diode=1e-3  Rs_Diode=1e6  Cs_Diode=inf  Vf_Diode=1e-3  Rs_CurrentSource=inf
      settings: SourceProductName=Simscape Electrical  SourceProductBaseCode=PS
  V DC : Scope  NumInputPorts=2
  Variables SC : Scope  NumInputPorts=3
  Variables SC1 : Scope  NumInputPorts=3
  VinvSC : Scope  NumInputPorts=2
  Voltage Measurement1 : powerlib/Measurements/Voltage Measurement  PhasorSimulation=off  OutputType=Complex  PSBequivalent=0
      settings: SourceProductName=Simscape Electrical
  A : PMIOPort  Side=Left
  B : PMIOPort  Port=2  Side=Left
  C : PMIOPort  Port=3  Side=Left
  wires:
  Current Measurement/1 -> [Isc_Meas]
  Bus Selector3/2 -> Variables SC/2, [VSC]  "<Voltage V>"
  Bus Selector3/3 -> [soc], Variables SC/3  "<SOC %>"
  Bus Selector3/1 -> Variables SC/1  "<Current I>"
  "Power (3ph, Instantaneous)2"/2 -> First-Order Filter4/1
  [Iabc_SC2] -> "Power (3ph, Instantaneous)2"/2
  First-Order Filter3/1 -> P SC in 1/1
  [Vabc_SC2] -> "Power (3ph, Instantaneous)2"/1
  First-Order Filter4/1 -> Q Sc in 1/1
  "Power (3ph, Instantaneous)2"/1 -> First-Order Filter3/1
  [Vabc_SC2] -> VinvSC/1
  Voltage Measurement1/1 -> [Vdc]
  [Uref] -> Two-Level Converter1/1
  Current Measurement1/1 -> [IoutConv]
  [Vdc] -> V DC/1
  [IoutConv] -> V DC/2
  Supercapacitor4/1 -> Bus Selector3/1
  Current Measurement2/1 -> Scope/1, [Iboost]
  [Iboost] -> Gain1/1
  Constant/1 -> Sum8/2
  [Vdc] -> Sum8/1
  Cast To Boolean1/1 -> S-R Flip-Flop/2
  Cast To Double/1 -> Mosfet/1
  Clock/1 -> Cast To Boolean/1
  Add/1 -> Switch/2
  Cast To Boolean/1 -> S-R Flip-Flop/1
  S-R Flip-Flop/1 -> Cast To Double/1
  Constant3/1 -> Switch/3
  Switch/1 -> Cast To Boolean1/1
  Constant2/1 -> Switch/1
  Sum8/1 -> PID Controller/1
  Bus Selector1/2 -> Variables SC1/2  "<Voltage (V)>"
  Battery/1 -> Bus Selector1/1
  Bus Selector1/3 -> Variables SC1/3  "<SOC (%)>"
  Bus Selector1/1 -> Variables SC1/1  "<Current (A)>"
  Gain1/1 -> Add/2
  PID Controller/1 -> Add/1
  Sawtooth Generator/1 -> Add1/1
  Add1/1 -> Gain/1
  Constant1/1 -> Add1/2
  Gain/1 -> Scope1/1
  connections:
  Current Measurement/RConn1 -- Series RLC Branch/LConn1
  Voltage Measurement1/LConn2 -- Battery/LConn2 -- Supercapacitor4/LConn2 -- Current Measurement2/RConn1 -- Two-Level Converter1/RConn2 -- Parallel RLC Branch/RConn1
  B/RConn1 -- Three-Phase V-I Measurement1/LConn2
  C/RConn1 -- Three-Phase V-I Measurement1/LConn3
  A/RConn1 -- Three-Phase V-I Measurement1/LConn1
  Parallel RLC Branch/LConn1 -- Two-Level Converter1/RConn1 -- Current Measurement1/RConn1 -- Voltage Measurement1/LConn1
  Diode/LConn1 -- Mosfet/LConn1 -- Current Measurement/LConn1
  Two-Level Converter1/LConn1 -- Three-Phase V-I Measurement1/RConn1
  Three-Phase V-I Measurement1/RConn2 -- Two-Level Converter1/LConn2
  Two-Level Converter1/LConn3 -- Three-Phase V-I Measurement1/RConn3
  Mosfet/RConn1 -- Current Measurement2/LConn1
  Diode/RConn1 -- Current Measurement1/LConn1
  Supercapacitor4/LConn1 -- Battery/LConn1 -- Series RLC Branch/RConn1

== system Modelo_Red_Mitigación_final/Modelo con compensación/Subsystem3/Subsystem2 ==
  AC_CONTROL ALGORITHM : Subsystem
  Battery : electricdrivelib/Extra Sources/Battery  BatType=Lithium-Ion  ShowTempParam=off  ThermalPreset=no  ShowAgeParam=off  NomV=1300  NomQ=1  SOC=80  Batt_Tr=2  PresetModel=off  MaxQ=1  MinV=1000  FullV=1500  Dis_rate=4000  R=0.01  Normal_OP=1  expZone="[1400     4.9130435]"  current=[0.2 0.4 1]  Units=Time  Tci=20  NomT=20  T2=-30  MaxQ2=4.8  FullV2=7.1  Normal_OP2=5.655  expZone2="[6.58           1]"  Rca=0.6  ti=2000  Dp=0  Neq0=0  Tsim=1e6  Ta1=25  Qeol=5.4*0.9  Reol=0.013333*1.2  Char_age=[2000, 3000]  Dis_age=[2000, 3000]  N1=1500  N2=10500  N3=1000  N4=1400  Ta2=45  N5=950
      settings: SourceProductName=Simscape Electrical
  Bus Selector1 : BusSelector  OutputSignals=Current (A),Voltage (V),SOC (%)
  Bus Selector3 : BusSelector  OutputSignals=Current I,Voltage V,SOC %
  Control1 : Subsystem
  "Control1 " : Subsystem  Commented=on
  Control2 : Subsystem  Commented=on
  Current Measurement{,1..4} (5 alike) : powerlib/Measurements/Current Measurement  PhasorSimulation=off  OutputType=Complex  PSBequivalent=0
      settings: SourceProductName=Simscape Electrical
  Currents : Scope  NumInputPorts=2
  First-Order Filter3 : powerlib_meascontrol/Filters/First-Order Filter  FilterType=Lowpass  Tc=10e-3  Ts=0  Initialize=on  Vac_Init=[0, 0, 60]  Vdc_Init=0  PlotResponse=off  FreqRange="[0,  200,  1]"
      settings: SourceProductName=Simscape Electrical
  First-Order Filter4 : powerlib_meascontrol/Filters/First-Order Filter  FilterType=Lowpass  Tc=10e-3  Ts=0  Initialize=on  Vac_Init=[0, 0, 60]  Vdc_Init=0  PlotResponse=off  FreqRange="[0,  200,  1]"
      settings: SourceProductName=Simscape Electrical
  Ground : powerlib/Elements/Ground  LConnTagsString=a
      settings: SourceProductName=Simscape Electrical
  Half-Bridge Converter : powerlib/Power Electronics/Half-Bridge Converter  Commented=on  ModelType=Switching devices  Ron=1e-3  Rs=1e6  Cs=inf  Vforward=[0,0]  Ron_Diode=1e-3  Rs_Diode=1e6  Cs_Diode=inf  Vf_Diode=1e-3  Rs_CurrentSource=inf
      settings: SourceProductName=Simscape Electrical  SourceProductBaseCode=PS
  Half-Bridge Converter1 : powerlib/Power Electronics/Half-Bridge Converter  ModelType=Switching devices  Ron=1e-3  Rs=1e6  Cs=inf  Vforward=[0,0]  Ron_Diode=1e-3  Rs_Diode=1e6  Cs_Diode=inf  Vf_Diode=1e-3  Rs_CurrentSource=inf
      settings: SourceProductName=Simscape Electrical  SourceProductBaseCode=PS
  Half-Bridge Converter2 : powerlib/Power Electronics/Half-Bridge Converter  ModelType=Switching devices  Ron=1e-3  Rs=1e6  Cs=inf  Vforward=[0,0]  Ron_Diode=1e-3  Rs_Diode=1e6  Cs_Diode=inf  Vf_Diode=1e-3  Rs_CurrentSource=inf
      settings: SourceProductName=Simscape Electrical  SourceProductBaseCode=PS
  P SC in 1 : Scope
  Parallel RLC Branch : powerlib/Elements/Parallel RLC Branch  LConnTagsString=a  RConnTagsString=__new0  BranchType=C  Resistance=0.01  Inductance=1e-3  SetiL0=off  InitialCurrent=0  Capacitance=220e-6  Setx0=on  InitialVoltage=1500  Measurements=None
      settings: SourceProductName=Simscape Electrical
  "Power (3ph, Instantaneous)2" : powerlib_meascontrol/Measurements/Power (3ph, Instantaneous)
      settings: SourceProductName=Simscape Electrical
  Q Sc in 1 : Scope
  Scope : Scope  NumInputPorts=3
  Series RLC Branch : powerlib/Elements/Series RLC Branch  LConnTagsString=__new0  RConnTagsString=__new0  BranchType=L  Resistance=65e-3  Inductance=416e-6  SetiL0=off  InitialCurrent=0  Capacitance=1e-6  Setx0=off  InitialVoltage=0  Measurements=None
      settings: SourceProductName=Simscape Electrical
  Series RLC Branch1 : powerlib/Elements/Series RLC Branch  LConnTagsString=__new0  RConnTagsString=__new0  BranchType=L  Resistance=65e-3  Inductance=1.67e-3  SetiL0=off  InitialCurrent=0  Capacitance=1e-6  Setx0=off  InitialVoltage=0  Measurements=None
      settings: SourceProductName=Simscape Electrical
  Supercapacitor4 : electricdrivelib/Extra Sources/Supercapacitor  C=5  Rdc=7e-3  Voltage=1000  Ns=1  Np=1  Vinit=1000  Temp=25  PresetModel=on  EstParam=off  Nc=1  r=1e-9  epsilon=6.0208e-10  Ich=10  Vstern="[0.161  2.7  7.8]"  Self_dis=off  Ioc=10  Vself="[48  47.8  47.06  44.65]"  demandeplot=off  I="[10  20 100  500]"  Units=sec  Vmax=0  If=0  deltaV=0  alpha=0  sec=0
      settings: SourceProductName=Simscape Electrical  SourceProductBaseCode=PS
  Three-Phase V-I Measurement1 : powerlib/Measurements/Three-Phase V-I Measurement  VoltageMeasurement=phase-to-phase  SetLabelV=on  LabelV=Vabc_SC2  Vpu=off  VpuLL=off  CurrentMeasurement=yes  SetLabelI=on  LabelI=Iabc_SC2  Ipu=off  Pbase=100e6  Vbase=500e3  OutputType=Complex  PhasorSimulation=off  PSBequivalent=0
      settings: SourceProductName=Simscape Electrical
  Two-Level Converter1 : powerlib/Power Electronics/Two-Level Converter  ModelType=Average model (Uref-controlled)  Ron=1e-3  Rs=1e6  Cs=inf  Vforward=[0,0]  Ron_Diode=1e-3  Rs_Diode=1e6  Cs_Diode=inf  Vf_Diode=1e-3  Rs_CurrentSource=inf
      settings: SourceProductName=Simscape Electrical  SourceProductBaseCode=PS
  V DC : Scope  NumInputPorts=2
  Variables SC : Scope  NumInputPorts=3
  Variables SC1 : Scope  NumInputPorts=3
  VinvSC : Scope  NumInputPorts=2
  Voltage Measurement : powerlib/Measurements/Voltage Measurement  PhasorSimulation=off  OutputType=Complex  PSBequivalent=0
      settings: SourceProductName=Simscape Electrical
  Voltage Measurement1 : powerlib/Measurements/Voltage Measurement  PhasorSimulation=off  OutputType=Complex  PSBequivalent=0
      settings: SourceProductName=Simscape Electrical
  A : PMIOPort  Side=Left
  B : PMIOPort  Port=2  Side=Left
  C : PMIOPort  Port=3  Side=Left
  tag scope: Ibat=global, Iload=global, Iobat=global, Iosc=global, Isc=global, Vdc=global
  wires:
  Bus Selector3/2 -> Variables SC/2, [VSC]  "<Voltage V>"
  Bus Selector3/3 -> [soc], Variables SC/3  "<SOC %>"
  Bus Selector3/1 -> Currents/1, Variables SC/1  "<Current I>"
  "Power (3ph, Instantaneous)2"/2 -> First-Order Filter4/1
  [Iabc_SC2] -> "Power (3ph, Instantaneous)2"/2
  First-Order Filter3/1 -> P SC in 1/1
  [Vabc_SC2] -> "Power (3ph, Instantaneous)2"/1
  First-Order Filter4/1 -> Q Sc in 1/1
  "Power (3ph, Instantaneous)2"/1 -> First-Order Filter3/1
  [Vabc_SC2] -> VinvSC/1
  [Uref] -> Two-Level Converter1/1
  [Vdc] -> V DC/1
  [IoutConv] -> V DC/2
  Supercapacitor4/1 -> Bus Selector3/1
  Bus Selector1/2 -> Variables SC1/2  "<Voltage (V)>"
  Battery/1 -> Bus Selector1/1
  Bus Selector1/3 -> Variables SC1/3  "<SOC (%)>"
  Bus Selector1/1 -> Currents/2, Variables SC1/1  "<Current (A)>"
  Current Measurement1/1 -> [Iload]
  Voltage Measurement/1 -> [Vdc]
  [G_BAT] -> Half-Bridge Converter2/1
  [G_SC] -> Half-Bridge Converter1/1
  Current Measurement3/1 -> [Iobat]
  Current Measurement4/1 -> [Iosc]
  [Iload] -> Scope/1  "Iload"
  [Iosc] -> Scope/2  "Isc"
  [Iobat] -> Scope/3  "Ibat"
  Current Measurement/1 -> [Isc]
  Current Measurement2/1 -> [Ibat]
  connections:
  B/RConn1 -- Three-Phase V-I Measurement1/LConn2
  C/RConn1 -- Three-Phase V-I Measurement1/LConn3
  A/RConn1 -- Three-Phase V-I Measurement1/LConn1
  Two-Level Converter1/LConn1 -- Three-Phase V-I Measurement1/RConn1
  Three-Phase V-I Measurement1/RConn2 -- Two-Level Converter1/LConn2
  Two-Level Converter1/LConn3 -- Three-Phase V-I Measurement1/RConn3
  Supercapacitor4/LConn1 -- Series RLC Branch/RConn1
  Current Measurement4/LConn1 -- Half-Bridge Converter1/RConn1
  Half-Bridge Converter2/RConn2 -- Ground/LConn1 -- Supercapacitor4/LConn2 -- Half-Bridge Converter1/RConn2 -- Voltage Measurement/LConn2 -- Parallel RLC Branch/RConn1 -- Two-Level Converter1/RConn2 -- Battery/LConn2 -- Voltage Measurement1/LConn2
  Series RLC Branch1/RConn1 -- Battery/LConn1 -- Voltage Measurement1/LConn1
  Current Measurement1/RConn1 -- Two-Level Converter1/RConn1
  Current Measurement3/LConn1 -- Half-Bridge Converter2/RConn1
  Current Measurement/LConn1 -- Series RLC Branch/LConn1
  Current Measurement/RConn1 -- Half-Bridge Converter1/LConn1
  Current Measurement2/LConn1 -- Series RLC Branch1/LConn1
  Current Measurement2/RConn1 -- Half-Bridge Converter2/LConn1
  Parallel RLC Branch/LConn1 -- Current Measurement3/RConn1 -- Voltage Measurement/LConn1 -- Current Measurement4/RConn1 -- Current Measurement1/LConn1
